simulink model "project_5"  (R2020a)
settings: Solver=VariableStepAuto  StartTime=0.0  StopTime=Sim_Time  RelTol=1e-3
values from neighbouring files (symbols this model uses):
  Cn = 2.3 * 3600    (= 8280)    [project_5m.m]
  I = 2.3    [project_5m.m]
  OCV = Data(:,2)    [project_5m.m]
  R_Charge = Data(:,3)    [project_5m.m]
  R_Discharge = Data(:,4)    [project_5m.m]
  SOC = Data(:,1)    [project_5m.m]
settings Model: Creator=Matt  LastModifiedBy=Matt
settings DataIOCC: ReturnWorkspaceOutputs=off

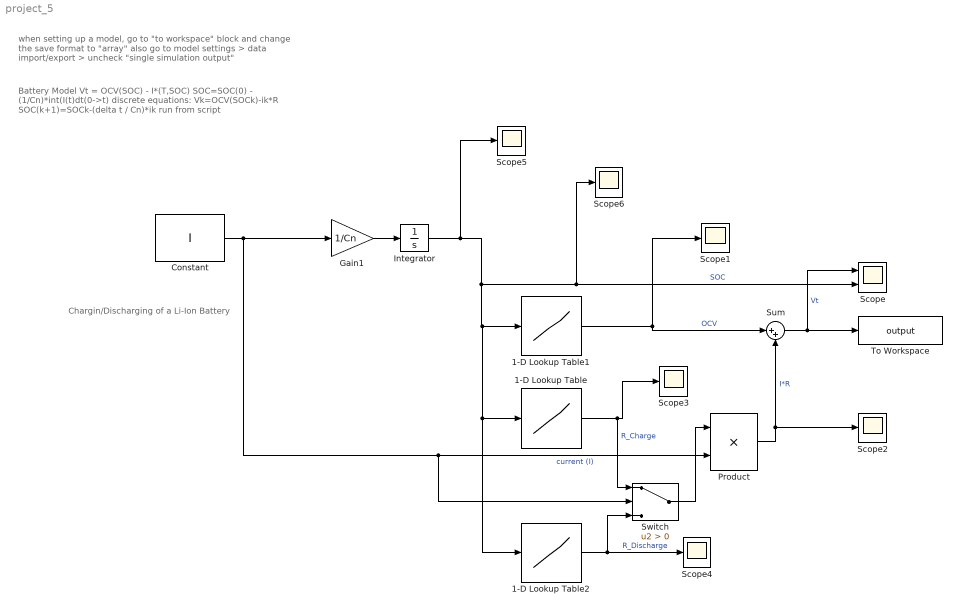
== system project_5 ==
  note: Chargin/Discharging of a Li-Ion Battery
  note: Battery Model
      | Vt = OCV(SOC) - I*(T,SOC)
      | SOC=SOC(0) - (1/Cn)*int(I(t)dt(0->t)
      | discrete equations:
      | Vk=OCV(SOCk)-ik*R
      | SOC(k+1)=SOCk-(delta t / Cn)*ik
      | run from script
  note: when setting up a model, go to "to workspace" block and change the save format to "array"
      | also go to model settings > data import/export > uncheck "single simulation output"
  1-D Lookup Table : Lookup_n-D  NumberOfTableDimensions=1  BreakpointsForDimension1=SOC  Table=R_Charge  InternalRulePriority=Speed  RndMeth=Simplest  InputSameDT=on
  1-D Lookup Table1 : Lookup_n-D  NumberOfTableDimensions=1  BreakpointsForDimension1=SOC  Table=OCV  InternalRulePriority=Speed  RndMeth=Simplest  InputSameDT=on
  1-D Lookup Table2 : Lookup_n-D  NumberOfTableDimensions=1  BreakpointsForDimension1=SOC  Table=R_Discharge  InternalRulePriority=Speed  RndMeth=Simplest  InputSameDT=on
  Constant : Constant  Value=I
  Gain1 : Gain  Gain=1/Cn
  Integrator : Integrator  InitialCondition=1
  Product : Product
  Scope : Scope  NumInputPorts=2
  Scope{1..6} (6 alike) : Scope
  Sum : Sum  Inputs=|++
  Switch : Switch  Criteria=u2 > Threshold
  To Workspace : ToWorkspace  VariableName=output  SampleTime=-1
  wires:
  Constant/1 -> Gain1/1, Switch/2, Product/2  "current (I)"
  Integrator/1 -> Scope6/1, Scope/2, 1-D Lookup Table2/1, 1-D Lookup Table/1, 1-D Lookup Table1/1, Scope5/1  "SOC"
  1-D Lookup Table/1 -> Switch/1, Scope3/1  "R_Charge"
  1-D Lookup Table1/1 -> Scope1/1, Sum/1  "OCV"
  Product/1 -> Scope2/1, Sum/2  "I*R"
  Sum/1 -> Scope/1, To Workspace/1  "Vt"
  1-D Lookup Table2/1 -> Switch/3, Scope4/1  "R_Discharge"
  Switch/1 -> Product/1
  Gain1/1 -> Integrator/1
